simulink model "Phase2_Section5_reduced"  (R2021b)
settings: Solver=VariableStepAuto  StartTime=0.0  StopTime=50.0  RelTol=1e-3
values from neighbouring files (symbols this model uses):
  A = [0 1 0; 244.86 -0.094 -26.29; 0 0 -250]    [Phase2_Section1.m]    (also in Phase2_Section2.m; Phase2_Section3.m; Phase2_Section4.m; Phase2_Section5.m)
  B = [0; 0; 5]    [Phase2_Section1.m]    (also in Phase2_Section2.m; Phase2_Section3.m; Phase2_Section4.m; Phase2_Section5.m)
  C = [1 0 0]    [Phase2_Section1.m]    (also in Phase2_Section2.m; Phase2_Section3.m; Phase2_Section4.m; Phase2_Section5.m)
  F = [-2 0; 0 -3]    [Phase2_Section5.m]
  F1 = P(:, 1)    [Phase2_Section5.m]
  F2 = P(:, 2:3)    [Phase2_Section5.m]
  K1 = place(A, B, p_fast)    [Phase2_Section1.m]    (also in Phase2_Section2.m; Phase2_Section3.m; Phase2_Section4.m = place(A, B, [-4 -2 -3]); Phase2_Section5.m = place(A, B, [-4 -2 -3]))
  L = [1;1]    [Phase2_Section5.m]
  T = lyap(-F,A,-L*C)    [Phase2_Section5.m]
settings Model: Creator=odeut  LastModifiedBy=odeut

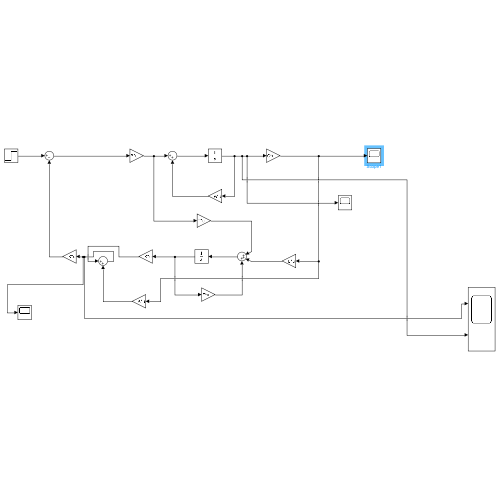
[thumbnail: Simulink's stored preview of the top-level diagram]
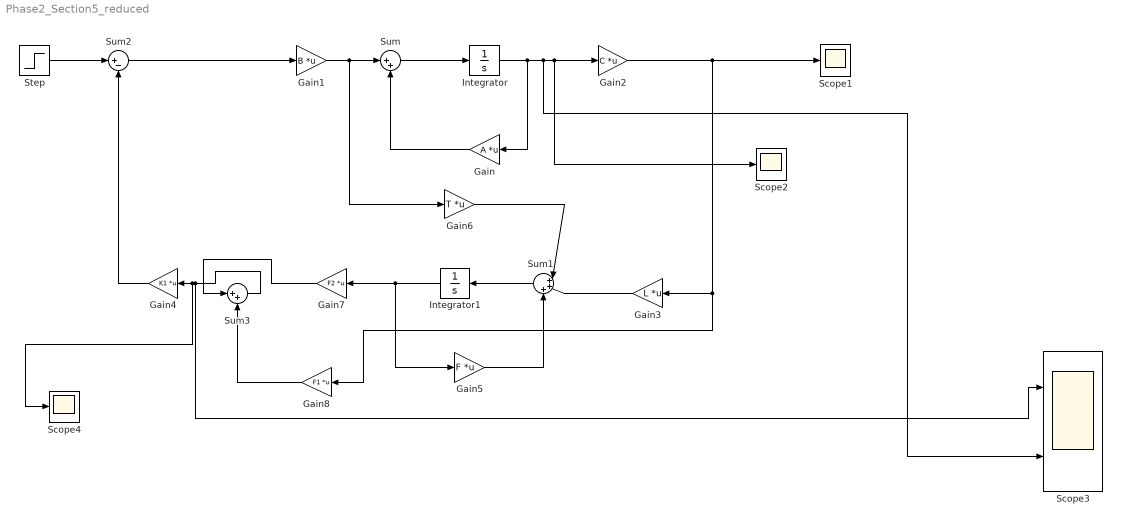
== system Phase2_Section5_reduced ==
  Gain : Gain  Gain=A  Multiplication=Matrix(K*u)
  Gain1 : Gain  Gain=B  Multiplication=Matrix(K*u)
  Gain2 : Gain  Gain=C  Multiplication=Matrix(K*u)
  Gain3 : Gain  Gain=L  Multiplication=Matrix(K*u)
  Gain4 : Gain  Gain=K1  Multiplication=Matrix(K*u)
  Gain5 : Gain  Gain=F  Multiplication=Matrix(K*u)
  Gain6 : Gain  Gain=T  Multiplication=Matrix(K*u)
  Gain7 : Gain  Gain=F2  Multiplication=Matrix(K*u)
  Gain8 : Gain  Gain=F1  Multiplication=Matrix(K*u)
  Integrator : Integrator
  Integrator1 : Integrator
  Scope1 : Scope
  Scope2 : Scope
  Scope3 : Scope  NumInputPorts=2
  Scope4 : Scope
  Step : Step  SampleTime=0
  Sum : Sum  Inputs=|++
  Sum1 : Sum  Inputs=|+++
  Sum2 : Sum  Inputs=|+-
  Sum3 : Sum  Inputs=|++
  wires:
  Gain6/1 -> Sum1/1
  Gain5/1 -> Sum1/3
  Sum/1 -> Integrator/1
  Gain2/1 -> Scope1/1, Gain8/1, Gain3/1
  Gain/1 -> Sum/2
  Sum2/1 -> Gain1/1
  Gain1/1 -> Gain6/1, Sum/1
  Gain3/1 -> Sum1/2
  Sum1/1 -> Integrator1/1
  Step/1 -> Sum2/1
  Integrator1/1 -> Gain7/1, Gain5/1
  Gain4/1 -> Sum2/2
  Gain8/1 -> Sum3/2
  Gain7/1 -> Sum3/1
  Sum3/1 -> Scope3/1, Scope4/1, Gain4/1
  Integrator/1 -> Scope3/2, Scope2/1, Gain2/1, Gain/1
